simulink model "mtv1_with_slosh_with_valve_delay"  (R2014b)
settings: Solver=ode4  SolverMode=SingleTasking  StartTime=0.0  StopTime=sim_stop_time  FixedStep=sim_time_step_size  RelTol=1e-3
PreLoadFcn:
  | nimbus_bus_all;
  | mtv_bus_all;
undefined symbols (not defined in the file or in its folder): csc_cnt_attitude_control, csc_cnt_attitude_control_lib, csc_cnt_dt, csc_egt_egc_thruster, csc_egt_egc_thruster_lib, csc_eom_six_dof_integration_fwdeuler, csc_eom_six_dof_integration_lib, csc_ppc_phase_plane_ctrl, csc_ppc_phase_plane_ctrl_lib, csc_rigid_body_dynamics, csc_rigid_body_dynamics_lib, csc_sim_mtv_simulation, csc_sim_mtv_simulation_lib, csc_thl_thrusters_mtv, csc_thl_thrusters_mtv_lib, csci_fsw_mtv, csci_fsw_mtv_lib, csci_gsse_mtv, csci_gsse_mtv_lib, csu_rrk_rotational_kinematics, csu_rrk_rotational_kinematics_lib, csu_rtk_translational_kinematics, csu_rtk_translational_kinematics_lib, csu_tpl_thruster_propellant_mtv, csu_tpl_thruster_propellant_mtv_lib, egt_feed_pressure, egt_g_times_isp, egt_pc_to_thrust_offset, egt_pc_to_thrust_slope, gdn_altitude_transition_free_drift_landing, gdn_altitude_transition_free_drift_takeoff, ini_epoch_seconds, ini_landed_flag, ini_thrust_to_weight_takeoff_limit, mpl_gn2_mass_initial, mpl_htp_mass_initial, ppc_coarse_thr_delay, ppc_fine_thr_delay, sim_time_step_size, swm_num_switches, tpl_coarse_acs_thrust_to_isp, tpl_egc_chamber_pressure_to_thrust, tpl_egc_throttle_to_mdot_gain, tpl_egc_throttle_to_thrust, tpl_egc_throttle_to_thrust_gain
libraries: util_common_lib x17, util_info_lib x13, util_quat_lib x8, simulink x8, csu_spv_simulated_press_valves_lib x4, csu_cfe_cfe_time_lib x2, csu_tlm_telemetry_lib x2, util_event_lib x2, util_frame_rotation_lib x2, csc_act_actuator_manager_mtv_lib x1, csc_cmp_command_mode_process_mtv_lib x1, util_extra_lib x1
(part 2 of 2)

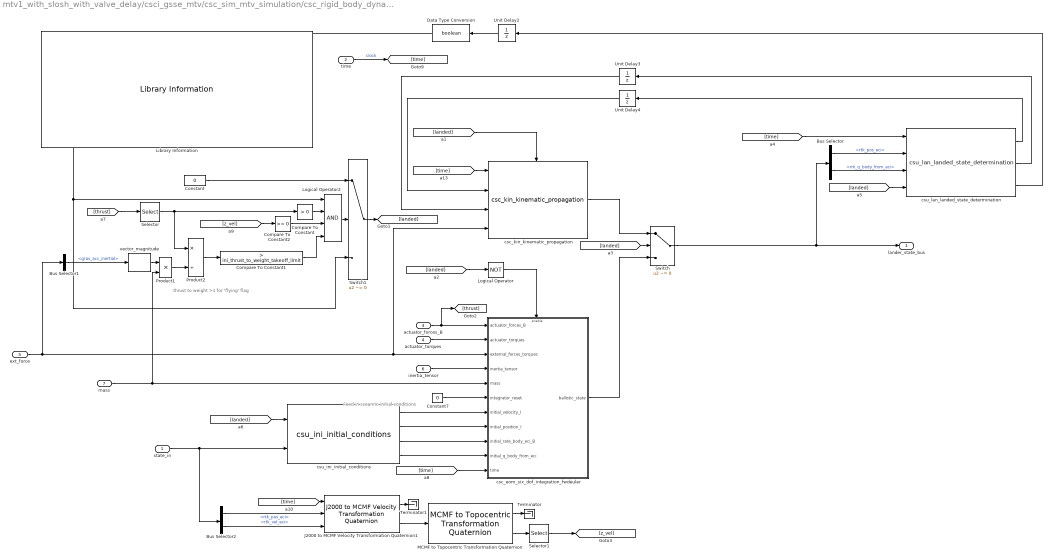
== system mtv1_with_slosh_with_valve_delay/csci_gsse_mtv/csc_sim_mtv_simulation/csc_rigid_body_dynamics ==
  note: thrust to weight >1 for
      | 'flying' flag
  note: Feed in sceanrio initial conditions
  state_in : Inport
  time : Inport  Port=2
  actuator_forces_B : Inport  Port=3
  actuator_torques : Inport  Port=4
  ext_force : Inport  Port=5
  inertia_tensor : Inport  Port=6
  mass : Inport  Port=7
  Bus Selector : BusSelector  OutputSignals=rtk_pos_eci,rrk_q_body_from_eci
  Bus Selector1 : BusSelector  OutputSignals=grav_acc_inertial
  Bus Selector2 : BusSelector  OutputSignals=rtk_pos_eci,rtk_vel_eci
  Compare To Constant : simulink/Logic and Bit Operations/Compare To Constant  relop=>  const=0  OutDataTypeStr=boolean
  Compare To Constant1 : simulink/Logic and Bit Operations/Compare To Constant  relop=>  const=ini_thrust_to_weight_takeoff_limit  OutDataTypeStr=boolean
  Compare To Constant2 : simulink/Logic and Bit Operations/Compare To Constant  relop=>=  const=0  OutDataTypeStr=boolean
  Constant : Constant  Value=0  OutDataTypeStr=boolean
  Constant7 : Constant  Value=0
  Data Type Conversion : DataTypeConversion  OutDataTypeStr=boolean
  J2000 to MCMF Velocity Transformation Quaternion1 : util_frame_rotation_lib/J2000 to MCMF Velocity Transformation Quaternion  SystemSampleTime=-1
  Library Information : util_info_lib/Library Information  owner='escrane'
  Logical Operator : Logic  Operator=NOT  AllPortsSameDT=off  OutDataTypeStr=boolean
  Logical Operator2 : Logic  Inputs=4  AllPortsSameDT=off  OutDataTypeStr=boolean
  MCMF to Topocentric Transformation Quaternion : util_frame_rotation_lib/MCMF to Topocentric  Transformation Quaternion  SystemSampleTime=-1
  Product1 : Product  RndMeth=Zero
  Product2 : Product  Inputs=*/  RndMeth=Zero
  Selector : Selector  InputPortWidth=3  Indices=3
  Selector1 : Selector  InputPortWidth=3  Indices=3
  Switch : Switch  Criteria=u2 ~= 0
  Switch1 : Switch  Criteria=u2 ~= 0
  Terminator : Terminator
  Terminator1 : Terminator
  Unit Delay2 : UnitDelay  InitialCondition=boolean(ini_landed_flag)  SampleTime=-1
  Unit Delay3 : UnitDelay  InitialCondition=[0 0 0 1]  SampleTime=-1
  Unit Delay4 : UnitDelay  InitialCondition=[0 0 0]  SampleTime=-1
  csc_eom_six_dof_integration_fwdeuler : Subsystem  AncestorBlock=csc_eom_six_dof_integration_lib/csc_eom_six_dof_integration_fwdeuler
  csc_kin_kinematic_propagation : csc_kin_kinematic_propagation_lib/csc_kin_kinematic_propagation
  csu_ini_initial_conditions : csu_ini_initial_conditions_lib/csu_ini_initial_conditions
  csu_lan_landed_state_determination : csu_lan_landed_state_determination_lib/csu_lan_landed_state_determination
  vector_magnitude : util_common_lib/vector_magnitude  SystemSampleTime=-1
  lander_state_bus : Outport
  wires:
  Switch1/1 -> [landed]
  actuator_torques/1 -> csc_eom_six_dof_integration_fwdeuler/2(actuator_torques)
  ext_force/1 -> csc_kin_kinematic_propagation/4, csc_eom_six_dof_integration_fwdeuler/3(external_forces_torques), Bus Selector1/1
  [time] -> csc_eom_six_dof_integration_fwdeuler/11(time)
  Data Type Conversion/1 -> Switch1/3, Logical Operator2/1
  Unit Delay2/1 -> Data Type Conversion/1
  Constant/1 -> Switch1/1
  Logical Operator2/1 -> Switch1/2
  [landed] -> csu_ini_initial_conditions/1
  Switch/1 -> Bus Selector/1, lander_state_bus/1
  time/1 -> [time]  "clock"
  csu_ini_initial_conditions/1 -> csc_eom_six_dof_integration_fwdeuler/7(initial_velocity_I)
  csu_ini_initial_conditions/2 -> csc_eom_six_dof_integration_fwdeuler/8(initial_position_I)
  csu_ini_initial_conditions/3 -> csc_eom_six_dof_integration_fwdeuler/9(initial_rate_body_eci_B)
  csu_ini_initial_conditions/4 -> csc_eom_six_dof_integration_fwdeuler/10(initial_q_body_from_eci)
  inertia_tensor/1 -> csc_eom_six_dof_integration_fwdeuler/4(inertia_tensor)
  Constant7/1 -> csc_eom_six_dof_integration_fwdeuler/6(integrator_reset)
  mass/1 -> csc_eom_six_dof_integration_fwdeuler/5(mass), Product1/2
  actuator_forces_B/1 -> [thrust], csc_eom_six_dof_integration_fwdeuler/1(actuator_forces_B)
  [time] -> csc_kin_kinematic_propagation/1
  [landed] -> csc_kin_kinematic_propagation/Enable
  [landed] -> Logical Operator/1
  [landed] -> Switch/2
  [time] -> csu_lan_landed_state_determination/1
  Bus Selector/1 -> csu_lan_landed_state_determination/2  "<rtk_pos_eci>"
  Bus Selector/2 -> csu_lan_landed_state_determination/3  "<rrk_q_body_from_eci>"
  [landed] -> csu_lan_landed_state_determination/4
  csu_lan_landed_state_determination/3 -> Unit Delay2/1
  Logical Operator/1 -> csc_eom_six_dof_integration_fwdeuler/Enable
  Bus Selector1/1 -> vector_magnitude/1  "<grav_acc_inertial>"
  Selector/1 -> Product2/1, Compare To Constant/1
  vector_magnitude/1 -> Product1/1
  Product1/1 -> Product2/2
  Compare To Constant/1 -> Logical Operator2/2
  Compare To Constant1/1 -> Logical Operator2/4
  Product2/1 -> Compare To Constant1/1
  csc_eom_six_dof_integration_fwdeuler/1(ballistic_state) -> Switch/3
  csc_kin_kinematic_propagation/1 -> Switch/1
  csu_lan_landed_state_determination/1 -> Unit Delay4/1
  csu_lan_landed_state_determination/2 -> Unit Delay3/1
  state_in/1 -> Bus Selector2/1, csu_ini_initial_conditions/2
  Unit Delay3/1 -> csc_kin_kinematic_propagation/3
  Unit Delay4/1 -> csc_kin_kinematic_propagation/2
  [thrust] -> Selector/1
  Bus Selector2/2 -> J2000 to MCMF Velocity Transformation Quaternion1/3  "<rtk_vel_eci>"
  MCMF to Topocentric Transformation Quaternion/2 -> Selector1/1
  Selector1/1 -> [z_vel]
  [z_vel] -> Compare To Constant2/1
  Compare To Constant2/1 -> Logical Operator2/3
  J2000 to MCMF Velocity Transformation Quaternion1/2 -> MCMF to Topocentric Transformation Quaternion/1
  MCMF to Topocentric Transformation Quaternion/1 -> Terminator/1
  J2000 to MCMF Velocity Transformation Quaternion1/1 -> Terminator1/1
  [time] -> J2000 to MCMF Velocity Transformation Quaternion1/1
  Bus Selector2/1 -> J2000 to MCMF Velocity Transformation Quaternion1/2  "<rtk_pos_eci>"

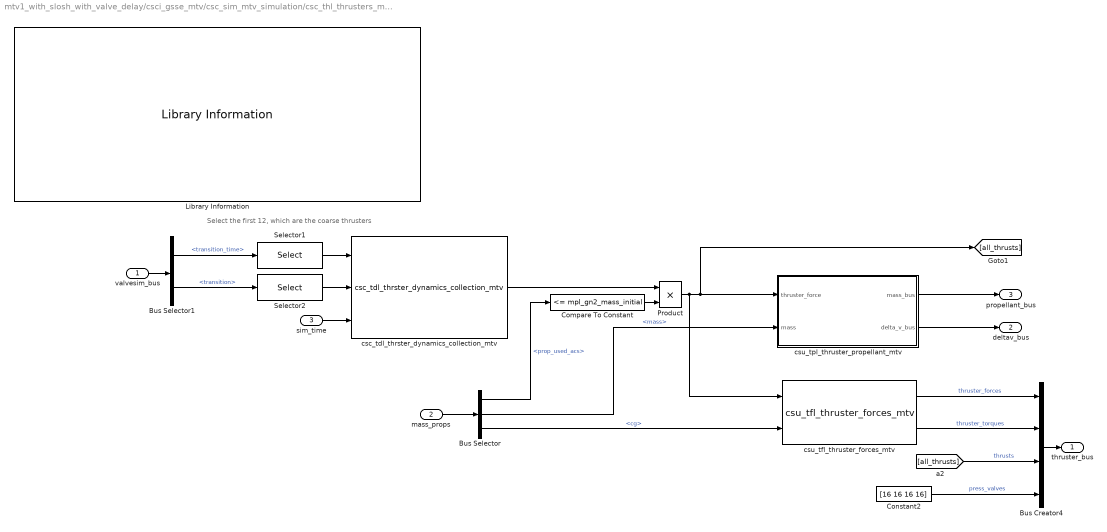
== system mtv1_with_slosh_with_valve_delay/csci_gsse_mtv/csc_sim_mtv_simulation/csc_thl_thrusters_mtv ==
  note: Select the first 12, which are the coarse thrusters
  valvesim_bus : Inport
  mass_props : Inport  Port=2
  sim_time : Inport  Port=3
  Bus Creator4 : BusCreator  OutDataTypeStr=Bus: actuator_mtv_msg_t
  Bus Selector : BusSelector  OutputSignals=prop_used_acs,mass,cg
  Bus Selector1 : BusSelector  OutputSignals=transition_time,transition
  Compare To Constant : simulink/Logic and Bit Operations/Compare To Constant  relop=<=  const=mpl_gn2_mass_initial  OutDataTypeStr=uint8
  Constant2 : Constant  Value=[16 16 16 16]  OutDataTypeStr=uint8
  Library Information : util_info_lib/Library Information  owner='NONE'
  Product : Product
  Selector1 : Selector  InputPortWidth=22  Indices=[1:12]
  Selector2 : Selector  InputPortWidth=22  Indices=[1:12]
  csc_tdl_thrster_dynamics_collection_mtv : csc_tdl_thruster_dynamics_collection_mtv_lib/csc_tdl_thrster_dynamics_collection_mtv  SystemSampleTime=-1
  csu_tfl_thruster_forces_mtv : csu_tfl_thruster_forces_mtv_lib/csu_tfl_thruster_forces_mtv
  csu_tpl_thruster_propellant_mtv : Subsystem  AncestorBlock=csu_tpl_thruster_propellant_mtv_lib/csu_tpl_thruster_propellant_mtv
  thruster_bus : Outport
  deltav_bus : Outport  Port=2
  propellant_bus : Outport  Port=3
  wires:
  Product/1 -> csu_tfl_thruster_forces_mtv/1, [all_thrusts], csu_tpl_thruster_propellant_mtv/1(thruster_force)
  mass_props/1 -> Bus Selector/1
  Bus Selector/2 -> csu_tpl_thruster_propellant_mtv/2(mass)  "<mass>"
  Bus Selector/3 -> csu_tfl_thruster_forces_mtv/2  "<cg>"
  sim_time/1 -> csc_tdl_thrster_dynamics_collection_mtv/3
  valvesim_bus/1 -> Bus Selector1/1
  csu_tpl_thruster_propellant_mtv/2(delta_v_bus) -> deltav_bus/1
  csu_tpl_thruster_propellant_mtv/1(mass_bus) -> propellant_bus/1
  Bus Selector1/2 -> Selector2/1  "<transition>"
  Bus Selector1/1 -> Selector1/1  "<transition_time>"
  Bus Creator4/1 -> thruster_bus/1
  csu_tfl_thruster_forces_mtv/2 -> Bus Creator4/2  "thruster_torques"
  csu_tfl_thruster_forces_mtv/1 -> Bus Creator4/1  "thruster_forces"
  [all_thrusts] -> Bus Creator4/3  "thrusts"
  csc_tdl_thrster_dynamics_collection_mtv/1 -> Product/1
  Compare To Constant/1 -> Product/2
  Selector1/1 -> csc_tdl_thrster_dynamics_collection_mtv/1
  Selector2/1 -> csc_tdl_thrster_dynamics_collection_mtv/2
  Bus Selector/1 -> Compare To Constant/1  "<prop_used_acs>"
  Constant2/1 -> Bus Creator4/4  "press_valves"

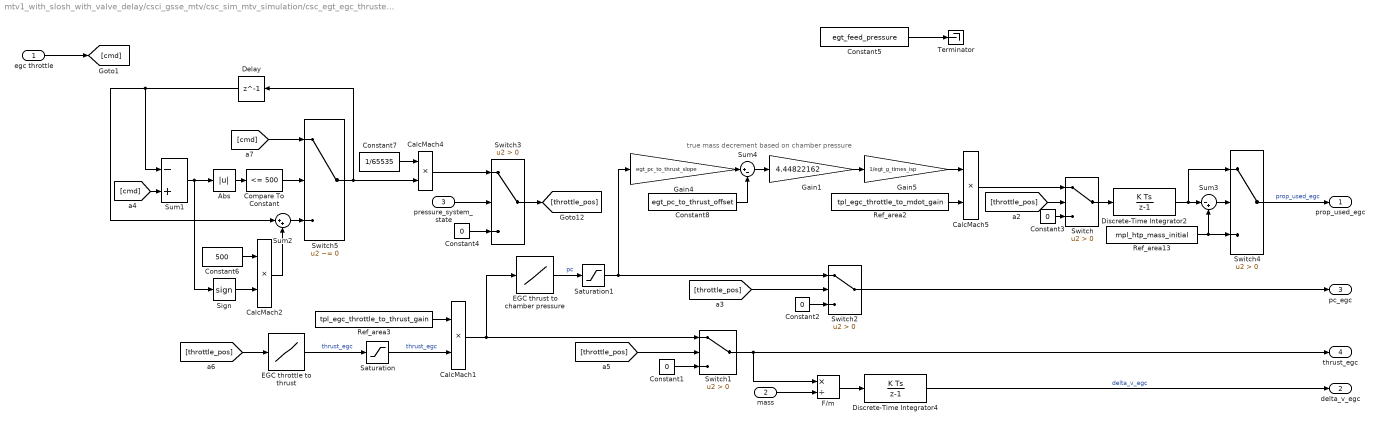
== system mtv1_with_slosh_with_valve_delay/csci_gsse_mtv/csc_sim_mtv_simulation/csc_egt_egc_thruster/EGC Forces, Delta-V and Propellant Usage ==
  note: true mass decrement based on chamber pressure
  egc throttle : Inport
  mass : Inport  Port=2
  pressure_system_state : Inport  Port=3
  Abs : Abs
  CalcMach{1..2,4..5} (4 alike) : Product  SaturateOnIntegerOverflow=on  OutDataTypeStr=Inherit: Same as first input
  Compare To Constant : simulink/Logic and Bit Operations/Compare To Constant  relop=<=  const=500  OutDataTypeStr=boolean
  Constant{1..4} (4 alike) : Constant  Value=0
  Constant5 : Constant  Value=egt_feed_pressure
  Constant6 : Constant  Value=500
  Constant7 : Constant  Value=1/65535
  Constant8 : Constant  Value=egt_pc_to_thrust_offset  OutDataTypeStr=double
  Delay : Delay  DelayLength=1
  Discrete-Time Integrator2 : DiscreteIntegrator  gainval=1  SampleTime=sim_time_step_size
  Discrete-Time Integrator4 : DiscreteIntegrator  gainval=1  SampleTime=sim_time_step_size
  "EGC thrust to chamber pressure " : Lookup  InputValues=tpl_egc_chamber_pressure_to_thrust(:,2)  Table=tpl_egc_chamber_pressure_to_thrust(:,1)
  EGC throttle to thrust : Lookup  InputValues=tpl_egc_throttle_to_thrust(:,1)  Table=tpl_egc_throttle_to_thrust(:,2)
  F/m : Product  Inputs=*/
  Gain1 : Gain  Gain=4.44822162
  Gain4 : Gain  Gain=egt_pc_to_thrust_slope
  Gain5 : Gain  Gain=1/egt_g_times_isp
  Ref_area13 : Constant  Value=mpl_htp_mass_initial
  Ref_area2 : Constant  Value=tpl_egc_throttle_to_mdot_gain
  Ref_area3 : Constant  Value=tpl_egc_throttle_to_thrust_gain
  Saturation : Saturate  UpperLimit=2300  LowerLimit=0
  Saturation1 : Saturate  UpperLimit=600  LowerLimit=0
  Sign : Signum
  Sum1 : Sum  Inputs=-+
  Sum2 : Sum  Inputs=|++
  Sum3 : Sum  Inputs=|-+
  Sum4 : Sum  Inputs=|+-
  Switch{,1..4} (5 alike) : Switch  Criteria=u2 > Threshold
  Switch5 : Switch  Criteria=u2 ~= 0
  Terminator : Terminator
  prop_used_egc : Outport
  delta_v_egc : Outport  Port=2
  pc_egc : Outport  Port=3
  thrust_egc : Outport  Port=4
  wires:
  CalcMach1/1 -> Switch1/1, "EGC thrust to chamber pressure "/1
  Switch2/1 -> pc_egc/1
  [throttle_pos] -> Switch2/2
  Constant2/1 -> Switch2/3
  Saturation/1 -> CalcMach1/2  "thrust_egc"
  [throttle_pos] -> Switch1/2
  Constant1/1 -> Switch1/3
  Switch1/1 -> F/m/1, thrust_egc/1
  Switch/1 -> Discrete-Time Integrator2/1
  [throttle_pos] -> Switch/2
  Constant3/1 -> Switch/3
  mass/1 -> F/m/2
  F/m/1 -> Discrete-Time Integrator4/1
  Switch4/1 -> prop_used_egc/1  "prop_used_egc"
  Discrete-Time Integrator4/1 -> delta_v_egc/1  "delta_v_egc"
  pressure_system_state/1 -> Switch3/2
  Constant4/1 -> Switch3/3
  Sum3/1 -> Switch4/2
  Discrete-Time Integrator2/1 -> Switch4/1, Sum3/1
  Ref_area13/1 -> Switch4/3, Sum3/2
  Constant5/1 -> Terminator/1
  Gain5/1 -> CalcMach5/1
  Ref_area3/1 -> CalcMach1/1
  egc throttle/1 -> [cmd]
  Delay/1 -> Sum1/1, Sum2/1
  Sum1/1 -> Sign/1, Abs/1
  Abs/1 -> Compare To Constant/1
  Compare To Constant/1 -> Switch5/2
  [cmd] -> Sum1/2
  [cmd] -> Switch5/1
  Switch5/1 -> CalcMach4/2, Delay/1
  Sum2/1 -> Switch5/3
  CalcMach2/1 -> Sum2/2
  Constant6/1 -> CalcMach2/1
  Sign/1 -> CalcMach2/2
  CalcMach4/1 -> Switch3/1
  Constant7/1 -> CalcMach4/1
  "EGC thrust to chamber pressure "/1 -> Saturation1/1  "pc"
  Sum4/1 -> Gain1/1
  Gain1/1 -> Gain5/1
  Gain4/1 -> Sum4/1
  Constant8/1 -> Sum4/2
  Switch3/1 -> [throttle_pos]
  [throttle_pos] -> EGC throttle to thrust/1
  EGC throttle to thrust/1 -> Saturation/1  "thrust_egc"
  Saturation1/1 -> Switch2/1, Gain4/1
  Ref_area2/1 -> CalcMach5/2
  CalcMach5/1 -> Switch/1

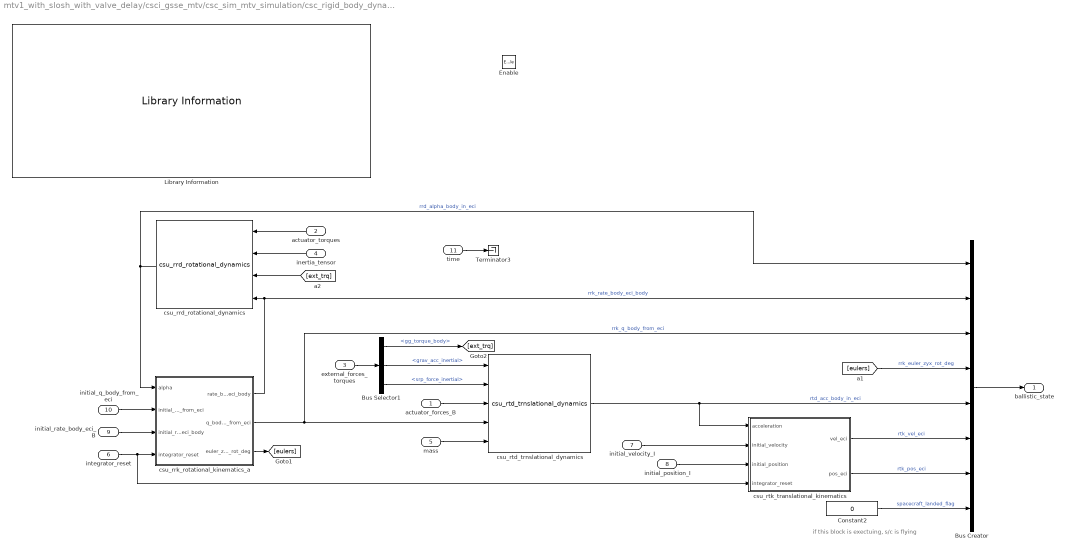
== system mtv1_with_slosh_with_valve_delay/csci_gsse_mtv/csc_sim_mtv_simulation/csc_rigid_body_dynamics/csc_eom_six_dof_integration_fwdeuler ==
  note: if this block is exectuing, s/c is flying
  actuator_forces_B : Inport
  actuator_torques : Inport  Port=2
  external_forces_torques : Inport  Port=3
  inertia_tensor : Inport  Port=4
  mass : Inport  Port=5
  integrator_reset : Inport  Port=6
  initial_velocity_I : Inport  Port=7
  initial_position_I : Inport  Port=8
  initial_rate_body_eci_B : Inport  Port=9
  initial_q_body_from_eci : Inport  Port=10
  time : Inport  Port=11
  Enable : EnablePort  StatesWhenEnabling=reset
  Bus Creator : BusCreator  Inputs=8  OutDataTypeStr=Bus: lander_state_bus_t
  Bus Selector1 : BusSelector  OutputSignals=gg_torque_body,grav_acc_inertial,srp_force_inertial
  Constant2 : Constant  Value=0
  Library Information : util_info_lib/Library Information  owner='escrane'
  Terminator3 : Terminator
  csu_rrd_rotational_dynamics : csu_rrd_rotational_dynamics_lib/csu_rrd_rotational_dynamics
  csu_rrk_rotational_kinematics_a : Subsystem  AncestorBlock=csu_rrk_rotational_kinematics_lib/csu_rrk_rotational_kinematics
  csu_rtd_trnslational_dynamics : csu_rtd_translational_dynamics_lib/csu_rtd_trnslational_dynamics
  csu_rtk_translational_kinematics : Subsystem  AncestorBlock=csu_rtk_translational_kinematics_lib/csu_rtk_translational_kinematics
  ballistic_state : Outport
  wires:
  time/1 -> Terminator3/1
  actuator_torques/1 -> csu_rrd_rotational_dynamics/1
  inertia_tensor/1 -> csu_rrd_rotational_dynamics/2
  initial_q_body_from_eci/1 -> csu_rrk_rotational_kinematics_a/2(initial_q_body_from_eci)
  initial_rate_body_eci_B/1 -> csu_rrk_rotational_kinematics_a/3(initial_rate_body_eci_body)
  integrator_reset/1 -> csu_rrk_rotational_kinematics_a/4(integrator_reset), csu_rtk_translational_kinematics/4(integrator_reset)
  mass/1 -> csu_rtd_trnslational_dynamics/5
  actuator_forces_B/1 -> csu_rtd_trnslational_dynamics/3
  initial_velocity_I/1 -> csu_rtk_translational_kinematics/2(initial_velocity)
  initial_position_I/1 -> csu_rtk_translational_kinematics/3(initial_position)
  csu_rrk_rotational_kinematics_a/3(euler_zyx_rot_deg) -> [eulers]
  csu_rtk_translational_kinematics/2(pos_eci) -> Bus Creator/7  "rtk_pos_eci"
  csu_rtk_translational_kinematics/1(vel_eci) -> Bus Creator/6  "rtk_vel_eci"
  csu_rtd_trnslational_dynamics/1 -> csu_rtk_translational_kinematics/1(acceleration), Bus Creator/5  "rtd_acc_body_in_eci"
  csu_rrk_rotational_kinematics_a/1(rate_body_eci_body) -> csu_rrd_rotational_dynamics/4, Bus Creator/2  "rrk_rate_body_eci_body"
  [eulers] -> Bus Creator/4  "rrk_euler_zyx_rot_deg"
  csu_rrd_rotational_dynamics/1 -> csu_rrk_rotational_kinematics_a/1(alpha), Bus Creator/1  "rrd_alpha_body_in_eci"
  csu_rrk_rotational_kinematics_a/2(q_body_from_eci) -> Bus Creator/3, csu_rtd_trnslational_dynamics/4  "rrk_q_body_from_eci"
  Bus Creator/1 -> ballistic_state/1
  external_forces_torques/1 -> Bus Selector1/1
  Bus Selector1/3 -> csu_rtd_trnslational_dynamics/2  "<srp_force_inertial>"
  Bus Selector1/1 -> [ext_trq]  "<gg_torque_body>"
  Bus Selector1/2 -> csu_rtd_trnslational_dynamics/1  "<grav_acc_inertial>"
  [ext_trq] -> csu_rrd_rotational_dynamics/3
  Constant2/1 -> Bus Creator/8  "spacecraft_landed_flag"

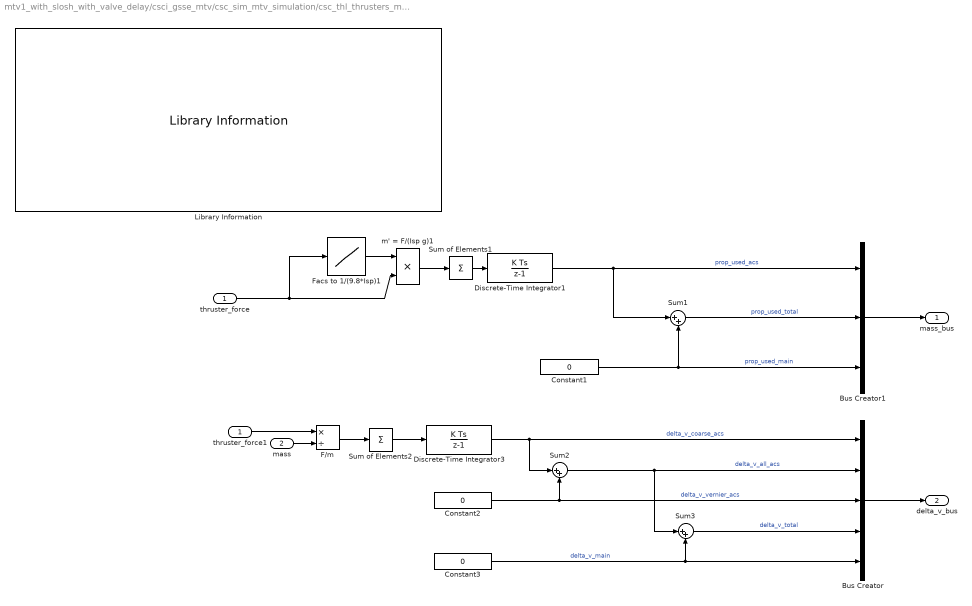
== system mtv1_with_slosh_with_valve_delay/csci_gsse_mtv/csc_sim_mtv_simulation/csc_thl_thrusters_mtv/csu_tpl_thruster_propellant_mtv ==
  thruster_force : Inport
  mass : Inport  Port=2
  Bus Creator : BusCreator  Inputs=5
  Bus Creator1 : BusCreator  Inputs=3
  Constant1 : Constant  Value=0  OutDataTypeStr=double
  Constant2 : Constant  Value=0  OutDataTypeStr=double
  Constant3 : Constant  Value=0  OutDataTypeStr=double
  Discrete-Time Integrator1 : DiscreteIntegrator  gainval=1  SampleTime=sim_time_step_size
  Discrete-Time Integrator3 : DiscreteIntegrator  gainval=1  SampleTime=sim_time_step_size
  F/m : Product  Inputs=*/
  Facs to 1/(9.8*Isp)1 : Lookup  InputValues=tpl_coarse_acs_thrust_to_isp(:,1)  Table=1./(9.8*tpl_coarse_acs_thrust_to_isp(:,2))  LookUpMeth=Interpolation-Use End Values
  Library Information : util_info_lib/Library Information  owner='escrane'
  Sum of Elements1 : Sum  Inputs=+
  Sum of Elements2 : Sum  Inputs=+
  Sum1 : Sum  Inputs=|++
  Sum2 : Sum  Inputs=|++
  Sum3 : Sum  Inputs=|++
  m' = F/(Isp g)1 : Product  RndMeth=Zero
  thruster_force1 : InportShadow
  mass_bus : Outport
  delta_v_bus : Outport  Port=2
  wires:
  Sum2/1 -> Sum3/1, Bus Creator/2  "delta_v_all_acs"
  Discrete-Time Integrator3/1 -> Sum2/1, Bus Creator/1  "delta_v_coarse_acs"
  Constant2/1 -> Sum2/2, Bus Creator/3  "delta_v_vernier_acs"
  Discrete-Time Integrator1/1 -> Sum1/1, Bus Creator1/1  "prop_used_acs"
  Sum1/1 -> Bus Creator1/2  "prop_used_total"
  m' = F/(Isp g)1/1 -> Sum of Elements1/1
  Facs to 1/(9.8*Isp)1/1 -> m' = F/(Isp g)1/1
  thruster_force/1 -> Facs to 1/(9.8*Isp)1/1, m' = F/(Isp g)1/2
  Sum of Elements1/1 -> Discrete-Time Integrator1/1
  Constant1/1 -> Sum1/2, Bus Creator1/3  "prop_used_main"
  mass/1 -> F/m/2
  F/m/1 -> Sum of Elements2/1
  Sum of Elements2/1 -> Discrete-Time Integrator3/1
  Sum3/1 -> Bus Creator/4  "delta_v_total"
  Constant3/1 -> Sum3/2, Bus Creator/5  "delta_v_main"
  Bus Creator/1 -> delta_v_bus/1
  Bus Creator1/1 -> mass_bus/1
  thruster_force1/1 -> F/m/1

== system mtv1_with_slosh_with_valve_delay/csci_gsse_mtv/csc_sim_mtv_simulation/csc_rigid_body_dynamics/csc_eom_six_dof_integration_fwdeuler/csu_rrk_rotational_kinematics_a ==
  alpha : Inport
  initial_q_body_from_eci : Inport  Port=2
  initial_rate_body_eci_body : Inport  Port=3
  integrator_reset : Inport  Port=4
  Constant1 : Constant  Value=0
  Discrete-Time Integrator1 : DiscreteIntegrator  ExternalReset=rising  InitialConditionSource=external  InitialConditionSetting=State (most efficient)  SampleTime=sim_time_step_size
  Library Information : util_info_lib/Library Information  owner='NONE'
  Sum : Sum  Inputs=|++
  quaternion_conjugate3 : util_quat_lib/quaternion_conjugate  SystemSampleTime=-1
  quaternion_propagator : Subsystem  AncestorBlock=util_quat_lib/quaternion_propagator
      mask Display:
      | disp('propogate(q)')
      | color('blue')
      | text(0.05,0.02,'NASA',...
      |  	'HorizontalAlignment','Left',...
      | 	'VerticalAlignment','bottom')
  quaternion_to_euler_angles (zyx) : util_quat_lib/quaternion_to_euler_angles (zyx)  SystemSampleTime=-1
  rad_to_deg : util_common_lib/rad_to_deg  SystemSampleTime=-1
  rate_body_eci_body : Outport
  q_body_from_eci : Outport  Port=2
  euler_zyx_rot_deg : Outport  Port=3
  wires:
  quaternion_propagator/1(quat) -> quaternion_conjugate3/1, q_body_from_eci/1  "rrk_q_body_from_eci"
  integrator_reset/1 -> quaternion_propagator/3(reset), Discrete-Time Integrator1/2
  Constant1/1 -> Discrete-Time Integrator1/3
  alpha/1 -> Discrete-Time Integrator1/1
  initial_rate_body_eci_body/1 -> Sum/1
  Discrete-Time Integrator1/1 -> Sum/2
  Sum/1 -> quaternion_propagator/2(omega), rate_body_eci_body/1  "rrk_rate_body_eci_body"
  initial_q_body_from_eci/1 -> quaternion_propagator/1(initial_q)
  quaternion_to_euler_angles (zyx)/1 -> rad_to_deg/1
  rad_to_deg/1 -> euler_zyx_rot_deg/1  "rrk_euler_zyx_rot_deg"
  quaternion_conjugate3/1 -> quaternion_to_euler_angles (zyx)/1

== system mtv1_with_slosh_with_valve_delay/csci_gsse_mtv/csc_sim_mtv_simulation/csc_rigid_body_dynamics/csc_eom_six_dof_integration_fwdeuler/csu_rtk_translational_kinematics ==
  acceleration : Inport
  initial_velocity : Inport  Port=2
  initial_position : Inport  Port=3
  integrator_reset : Inport  Port=4
  Constant1 : Constant  Value=0
  Constant2 : Constant  Value=0
  Discrete-Time Integrator1 : DiscreteIntegrator  ExternalReset=rising  InitialConditionSource=external  InitialConditionSetting=State (most efficient)  SampleTime=sim_time_step_size
  Discrete-Time Integrator2 : DiscreteIntegrator  ExternalReset=rising  InitialConditionSource=external  InitialConditionSetting=State (most efficient)  SampleTime=sim_time_step_size
  Library Information : util_info_lib/Library Information  owner='NONE'
  Sum : Sum  Inputs=++|
  Sum1 : Sum  Inputs=|++
  vel_eci : Outport
  pos_eci : Outport  Port=2
  wires:
  initial_position/1 -> Sum1/2
  Sum1/1 -> pos_eci/1  "rtk_pos_eci"
  Constant1/1 -> Discrete-Time Integrator2/3
  Sum/1 -> Discrete-Time Integrator2/1, vel_eci/1  "rtk_vel_eci"
  acceleration/1 -> Discrete-Time Integrator1/1
  Constant2/1 -> Discrete-Time Integrator1/3
  initial_velocity/1 -> Sum/1
  Discrete-Time Integrator2/1 -> Sum1/1
  Discrete-Time Integrator1/1 -> Sum/2
  integrator_reset/1 -> Discrete-Time Integrator2/2, Discrete-Time Integrator1/2

== system mtv1_with_slosh_with_valve_delay/csci_gsse_mtv/csc_sim_mtv_simulation/csc_rigid_body_dynamics/csc_eom_six_dof_integration_fwdeuler/csu_rrk_rotational_kinematics_a/quaternion_propagator ==
  initial_q : Inport
  omega : Inport  Port=2
  reset : Inport  Port=3
  Constant1 : Constant  Value=0
  Discrete-Time Integrator1 : DiscreteIntegrator  ExternalReset=rising  InitialConditionSource=external  SampleTime=sim_time_step_size
  Library Information : util_info_lib/Library Information  owner='NONE'
  Sum1 : Sum  Inputs=|++
  quaternion_derivative : util_quat_lib/quaternion_derivative  SystemSampleTime=-1
  unit_vector : util_common_lib/unit_vector  SystemSampleTime=-1
  quat : Outport
  wires:
  omega/1 -> quaternion_derivative/1
  unit_vector/1 -> quaternion_derivative/2, quat/1
  quaternion_derivative/1 -> Discrete-Time Integrator1/1
  Sum1/1 -> unit_vector/1
  reset/1 -> Discrete-Time Integrator1/2
  initial_q/1 -> Sum1/1
  Discrete-Time Integrator1/1 -> Sum1/2
  Constant1/1 -> Discrete-Time Integrator1/3
